simulink model "aTestModel"  (R2015b)
settings: Solver=ode45  StartTime=0.0  StopTime=2  RelTol=1e-6
values from neighbouring files (symbols this model uses):
  B_f = 7.7e-3    (= 0.0077)    [aTestComparison.m]    (also in aTestComparisonOLD.m)
  g = 9.82    [aTestComparison.m]    (also in aTestComparisonOLD.m)
  J_f = 4.8e-3    (= 0.0048)    [aTestComparison.m]    (also in aTestComparisonOLD.m)
  J_w = 0.601e-3    (= 0.000601)    [aTestComparison.m]    (also in aTestComparisonOLD.m)
  l_f = 0.08498    [aTestComparison.m]    (also in aTestComparisonOLD.m = 0.076)
  l_w = 0.093    [aTestComparison.m]    (also in aTestComparisonOLD.m)
  m_f = 0.77-m_w    (= 0.548)    [aTestComparison.m]    (also in aTestComparisonOLD.m = 0.354)
  m_w = 0.222    [aTestComparison.m]    (also in aTestComparisonOLD.m)
settings Model: Creator=USUARIO  LastModifiedBy=USUARIO
settings DataIOCC: LimitDataPoints=off  SaveFormat=Array
settings DebuggingCC: SolverPrmCheckMsg=warning
settings HardwareCC: ProdBitPerPointer=32  ProdLargestAtomicFloat=None  ProdIntDivRoundTo=Undefined  ProdEndianess=Unspecified  ProdWordSize=32  ProdHWDeviceType=32-bit Generic
settings GRTTargetCC: GeneratePreprocessorConditionals=Disable all
settings ConfigComp: CovModelRefEnable=Off  CovSFcnEnable=off

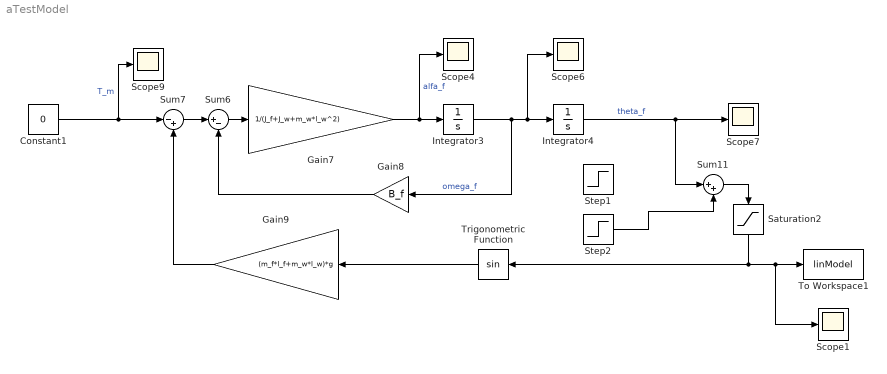
== system aTestModel ==
  Constant1 : Constant  Value=0
  Gain7 : Gain  Gain=1/(J_f+J_w+m_w*l_w^2)
  Gain8 : Gain  Gain=B_f
  Gain9 : Gain  Gain=(m_f*l_f+m_w*l_w)*g
  Integrator3 : Integrator
  Integrator4 : Integrator
  Saturation2 : Saturate  UpperLimit=0.85  LowerLimit=-0.72
  Scope{1,4,6..7,9} (5 alike) : Scope
  Step1 : Step  Time=0.0001  Before=-0.001  After=0  SampleTime=0
  Step2 : Step  Time=0  After=-0.14  SampleTime=0
  Sum11 : Sum  Inputs=|++
  Sum6 : Sum  Inputs=|+-
  Sum7 : Sum  Inputs=|-+
  To Workspace1 : ToWorkspace  VariableName=linModel  SaveFormat=Timeseries  SampleTime=-1
  Trigonometric Function : Trigonometry
  wires:
  Gain7/1 -> Scope4/1, Integrator3/1  "alfa_f"
  Integrator3/1 -> Gain8/1, Scope6/1, Integrator4/1  "omega_f"
  Sum6/1 -> Gain7/1
  Sum7/1 -> Sum6/1
  Gain8/1 -> Sum6/2
  Gain9/1 -> Sum7/2
  Constant1/1 -> Sum7/1, Scope9/1  "T_m"
  Integrator4/1 -> Scope7/1, Sum11/1  "theta_f"
  Sum11/1 -> Saturation2/1
  Saturation2/1 -> Trigonometric Function/1, Scope1/1, To Workspace1/1
  Trigonometric Function/1 -> Gain9/1
  Step2/1 -> Sum11/2
